simulink model "model_1"  (R2024a)
settings: Solver=ode45  StartTime=0.0  StopTime=20  MaxStep=0.01  RelTol=1e-5  AbsTol=1e-5
values from neighbouring files (symbols this model uses):
  A = [8 1 11 ... (first row only)    [init.m]
  B = [-1; -3; 3]    [init.m]
  B_f = [1, -1 ... (first row only)    [init.m]
  bool_K = 1    [init.m]
  bool_K_f = 1    [init.m]
  bool_K_g = 1    [init.m]
  C = [-2 0 -3]    [init.m]
  D = 15    [init.m]
  D_f = [0 3]    [init.m]
  G_f = [35 10 -28 17 ... (first row only)    [init.m]
  G_g = [0 0 0 ... (first row only)    [init.m]
  K = [-3.5 1 -3.5]    [init.m]
  K_f = [4.67331092826515         0.939042762776683         -2.71036315323295         -1.34100974313552]    [init.m]    (also in tester.m = [real(Kf_complex(1)), imag(Kf_complex(1)), real(Kf_complex(3)
  K_g = [0.0703124999999999       -0.0561558901682905        0.0658104517271922]    [init.m]    (also in tester.m = [real(Kg0), real(Kg2), imag(Kg2)])
  wf0 = [1; 1; 1; 1]    [init.m]
  wg0 = [-12; 0; 21]    [init.m]
  x0 = [0; 0; 0]    [init.m]
  Y_f = [12 -6 ... (first row only)    [init.m]
  Y_g = [1, 1, 0]    [init.m]
settings Model: Creator=eva  LastModifiedBy=eva

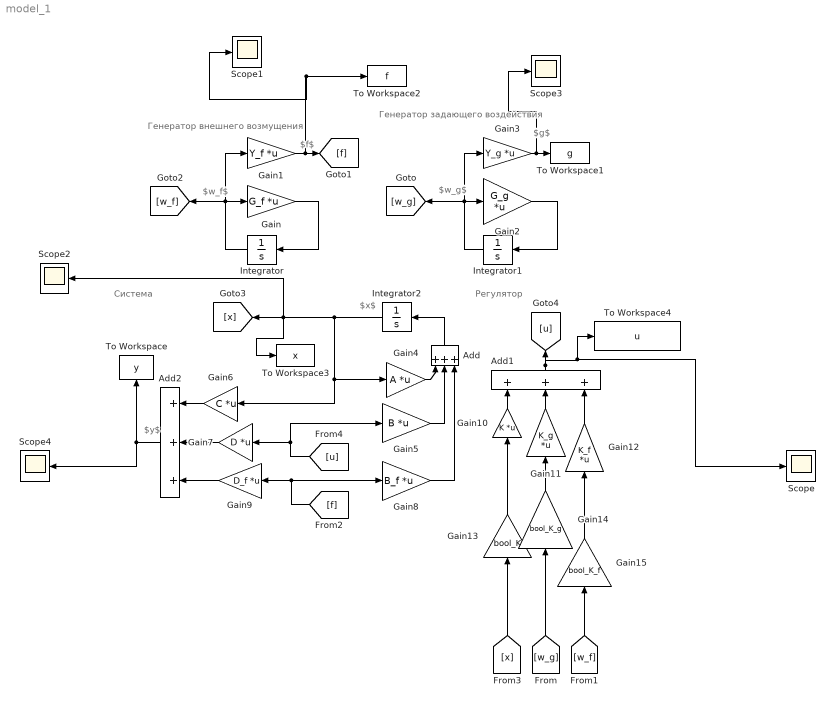
== system model_1 ==
  note: Система
  note: Регулятор
  note: Генератор задающего воздействия
  note: Генератор внешнего возмущения
  note: $x$
  note: $w_f$
  note: $f$
  note: $w_g$
  note: $g$
  note: $y$
  Add : Sum  Inputs=+++
  Add1 : Sum  Inputs=+++
  Add2 : Sum  Inputs=+++
  Gain : Gain  Gain=G_f  Multiplication=Matrix(K*u)
  Gain1 : Gain  Gain=Y_f  Multiplication=Matrix(K*u)
  Gain10 : Gain  Gain=K  Multiplication=Matrix(K*u)
  Gain11 : Gain  Gain=K_g  Multiplication=Matrix(K*u)
  Gain12 : Gain  Gain=K_f  Multiplication=Matrix(K*u)
  Gain13 : Gain  Gain=bool_K
  Gain14 : Gain  Gain=bool_K_g
  Gain15 : Gain  Gain=bool_K_f
  Gain2 : Gain  Gain=G_g  Multiplication=Matrix(K*u)
  Gain3 : Gain  Gain=Y_g  Multiplication=Matrix(K*u)
  Gain4 : Gain  Gain=A  Multiplication=Matrix(K*u)
  Gain5 : Gain  Gain=B  Multiplication=Matrix(K*u)
  Gain6 : Gain  Gain=C  Multiplication=Matrix(K*u)
  Gain7 : Gain  Gain=D  Multiplication=Matrix(K*u)
  Gain8 : Gain  Gain=B_f  Multiplication=Matrix(K*u)
  Gain9 : Gain  Gain=D_f  Multiplication=Matrix(K*u)
  Integrator : Integrator  InitialCondition=wf0
  Integrator1 : Integrator  InitialCondition=wg0
  Integrator2 : Integrator  InitialCondition=x0
  Scope{,1..4} (5 alike) : Scope
  To Workspace : ToWorkspace  VariableName=y  SaveFormat=Structure With Time  SampleTime=-1
  To Workspace1 : ToWorkspace  VariableName=g  SaveFormat=Structure With Time  SampleTime=-1
  To Workspace2 : ToWorkspace  VariableName=f  SaveFormat=Structure With Time  SampleTime=-1
  To Workspace3 : ToWorkspace  VariableName=x  SaveFormat=Structure With Time  SampleTime=-1
  To Workspace4 : ToWorkspace  VariableName=u  SaveFormat=Structure With Time  SampleTime=-1
  wires:
  Integrator/1 -> Gain/1, Gain1/1, [w_f]
  Gain/1 -> Integrator/1
  Gain2/1 -> Integrator1/1
  Gain3/1 -> Scope3/1, To Workspace1/1
  Integrator1/1 -> Gain2/1, [w_g], Gain3/1
  Gain4/1 -> Add/1
  Gain5/1 -> Add/2
  Add/1 -> Integrator2/1
  [u] -> Gain5/1, Gain7/1
  Gain8/1 -> Add/3
  Add2/1 -> Scope4/1, To Workspace/1
  [f] -> Gain9/1, Gain8/1
  Gain9/1 -> Add2/3
  Gain7/1 -> Add2/2
  Gain6/1 -> Add2/1
  Integrator2/1 -> Gain6/1, Gain4/1, Scope2/1, To Workspace3/1, [x]
  Gain10/1 -> Add1/1
  Gain11/1 -> Add1/2
  Gain12/1 -> Add1/3
  Add1/1 -> Scope/1, To Workspace4/1, [u]
  Gain1/1 -> Scope1/1, To Workspace2/1, [f]
  [w_f] -> Gain15/1
  Gain15/1 -> Gain12/1
  [w_g] -> Gain14/1
  Gain14/1 -> Gain11/1
  [x] -> Gain13/1
  Gain13/1 -> Gain10/1
